simulink model "digiex3"  (R2017b)
settings: Solver=ode23tb  StartTime=0.0  StopTime=15  RelTol=1e-3
values from neighbouring files (symbols this model uses):
  AT_gain = ones(1,N)    [parameter_project.m]
  ctrl_mtrx2 = combvec(ctrl_mtrx',ctrl_mtrx')'    [parameter_project.m]
  DFCU_AT_REAL = DFCU.AT_Kv.*(1+0.2*(rand(1,N)-0.5))    [parameter_project.m]
  DFCU_PA_REAL = DFCU.PA_Kv.*(1+0.2*(rand(1,N)-0.5))    [parameter_project.m]
  Kff = 1    [User_interface.m]
  Kp = 10    [User_interface.m]
  Kv = 2.5e-7    (= 2.5e-07)    [parameter_project.m]
  PA_gain = ones(1,N)    [parameter_project.m]
  ptr = 1e5    (= 100000)    [parameter_project.m]
  switch_gain = 5e-2    (= 0.05)    [User_interface.m]
  ts = 0.01    [parameter_project.m]
undefined symbols (not defined in the file or in its folder): Controller, Cyl, DFCU, Fric, Load, Supply, Tank, Valve
libraries: dspmtrx3 x2, dspstat3 x1
settings Model: Creator=ganguly  LastModifiedBy=pallab
settings CodeAppCC: StateflowObjectComments=on
settings SimscapeCC: SimscapeNormalizeSystem=off

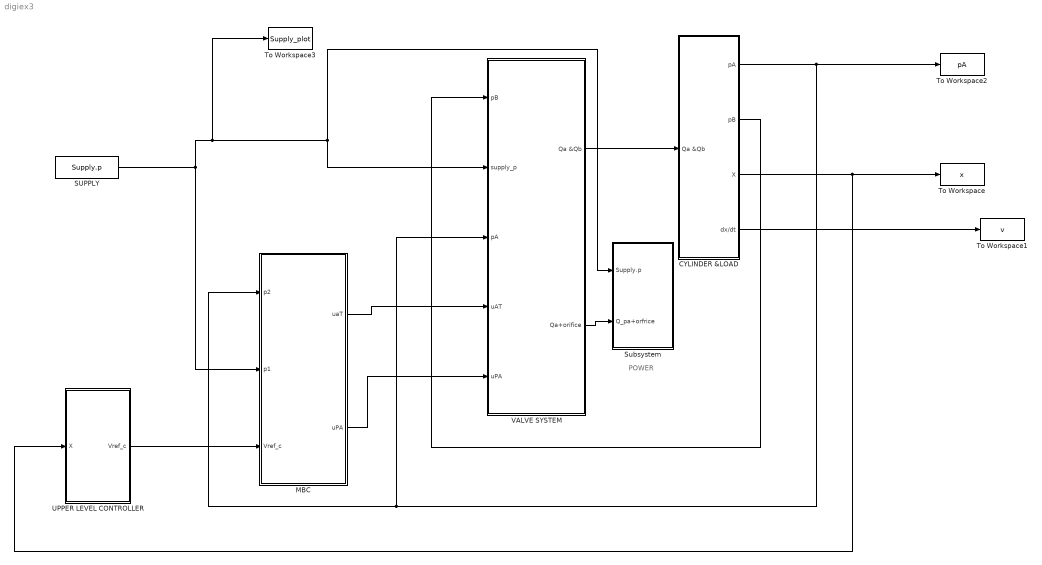
== system digiex3 ==
  note: POWER
  CYLINDER &LOAD : Subsystem
  MBC : Subsystem
  SUPPLY : Constant  Value=Supply.p
  Subsystem : Subsystem
  To Workspace : ToWorkspace  VariableName=x  SampleTime=-1
  To Workspace1 : ToWorkspace  VariableName=v  SampleTime=-1
  To Workspace2 : ToWorkspace  VariableName=pA  SampleTime=-1
  To Workspace3 : ToWorkspace  VariableName=Supply_plot  SampleTime=-1
      settings: Save2DSignal=2-D array (concatenate along first dimension)
  UPPER LEVEL CONTROLLER : Subsystem
  VALVE SYSTEM : Subsystem
  wires:
  SUPPLY/1 -> MBC/2(p1), To Workspace3/1, VALVE SYSTEM/2(supply_p), Subsystem/1(Supply.p)
  UPPER LEVEL CONTROLLER/1(Vref_c) -> MBC/3(Vref_c)
  CYLINDER &LOAD/3(X) -> UPPER LEVEL CONTROLLER/1(X), To Workspace/1
  CYLINDER &LOAD/1(pA) -> MBC/1(p2), VALVE SYSTEM/3(pA), To Workspace2/1
  VALVE SYSTEM/1(Qa &Qb) -> CYLINDER &LOAD/1(Qa &Qb)
  CYLINDER &LOAD/2(pB) -> VALVE SYSTEM/1(pB)
  CYLINDER &LOAD/4(dx/dt) -> To Workspace1/1
  MBC/2(uPA) -> VALVE SYSTEM/5(uPA)
  MBC/1(uaT) -> VALVE SYSTEM/4(uAT)
  VALVE SYSTEM/2(Qa+orifice) -> Subsystem/2(Q_pa+orfrice)

== system digiex3/CYLINDER &LOAD ==
  Qa &Qb : Inport
  Cylinder : Subsystem  mask(Hydraulic){D=[Cyl.D Cyl.d], xmax=Cyl.x_max, Vdead=[1e-4  1e-4], Vhose=[0 0], B_o=Cyl.B, Bhose=[400e6 400e6], pini=[Cyl.pA_init   Cyl.pB_init]}
      mask prompts: D "Diameters of piston and piston rod [m  m] :"; xmax "Cylindes stroke [m] :"; Vdead "Dead volumes at cylinder ends [m^3  m^3] :"; Vhose "Volumes of hoses [m^3  m^3] :"; B_o "Bulk modulus of oil [Pa] :"; Bhose "Bulk moduli of hoses [Pa  Pa] :"; pini "Initial pressures [Pa Pa] :"
      mask init:
      | A_A = pi/4*D(1)^2; A_B = A_A-pi/4*D(2)^2; V_0A = Vdead(1); V_0B = Vdead(2); V_HA = Vhose(1); V_HB = Vhose(2); B_HA = Bhose(1); B_HB = Bhose(2); p_0A = pini(1); p_0B = pini(2);
  Demux : Demux  Outputs=2
  Single mass model with friction and ends : Subsystem  mask(Mechanism){m=Load.m, range=[0, Cyl.x_max], xini=Cyl.x_init, Fricparams=[Fric.Fs  Fric.Fc  Fric.b  Fric.vtol Fric.m_est], presl=Fric.preslide, Kj=Cyl.End_K, g=-9.8}
      mask prompts: m "Mass [kg] :"; range "Range of motion [m  m] :"; xini "Initial position [m] :"; Fricparams "Friction parameters [Fs, Fc, b, vtol, mest]:"; presl "Pre-sliding displacement [m] :"; Kj "Spring constant of end [N/m] :"; g "gravity [m/s^2]"
      mask help:
      | Mechanism for linear movenment.
      | Model includes:
      | Inertia: F = m*a
      | Friction: Dynamic friction model (cf.IHA-2600)
      | End Springs: Use high spring constant and stiff solver for realistic results
      | Gravity: 0 if horizontal path, g if vertical. Careful with sign! (Look under mask)
      mask init:
      | xmax=range(2);xmin=range(1);
  pA : Outport
  pB : Outport  Port=2
  X : Outport  Port=3
  dx/dt : Outport  Port=4
  wires:
  Single mass model with friction and ends/1(x) -> X/1, Cylinder/2(x)
  Qa &Qb/1 -> Cylinder/1(QA & QB)
  Demux/2 -> pB/1
  Single mass model with friction and ends/2(dx/dt) -> dx/dt/1, Cylinder/3(dx/dt)
  Cylinder/1(pA & pB) -> Demux/1
  Cylinder/2(F) -> Single mass model with friction and ends/1(F)
  Demux/1 -> pA/1

== system digiex3/MBC ==
  p2 : Inport
  p1 : Inport  Port=2
  Vref_c : Inport  Port=3
  Constant1 : Constant  Value=Tank.p
  Gain2 : Gain  Gain=Cyl.area
  Gain4 : Gain  Gain=1/Cyl.area
  To Workspace : ToWorkspace  VariableName=v_est  SampleTime=-1
      settings: Save2DSignal=2-D array (concatenate along first dimension)
  mbc_PA : Subsystem
  uaT : Outport
  uPA : Outport  Port=2
  wires:
  mbc_PA/1(Q_estimate) -> Gain4/1
  p2/1 -> mbc_PA/3(pA1)
  Gain2/1 -> mbc_PA/1(Q_ref)
  mbc_PA/3(uaT) -> uaT/1
  Gain4/1 -> To Workspace/1
  mbc_PA/2(uPA) -> uPA/1
  p1/1 -> mbc_PA/2(pP)
  Vref_c/1 -> mbc_PA/5(V_ref), Gain2/1
  Constant1/1 -> mbc_PA/4(pT)

== system digiex3/Subsystem ==
  Supply.p : Inport
  Q_pa+orfrice : Inport  Port=2
  Gain1 : Gain  Gain=-1
  Product : Product
  To Workspace : ToWorkspace  VariableName=power  SampleTime=-1
  wires:
  Q_pa+orfrice/1 -> Product/2
  Supply.p/1 -> Product/1
  Product/1 -> Gain1/1
  Gain1/1 -> To Workspace/1

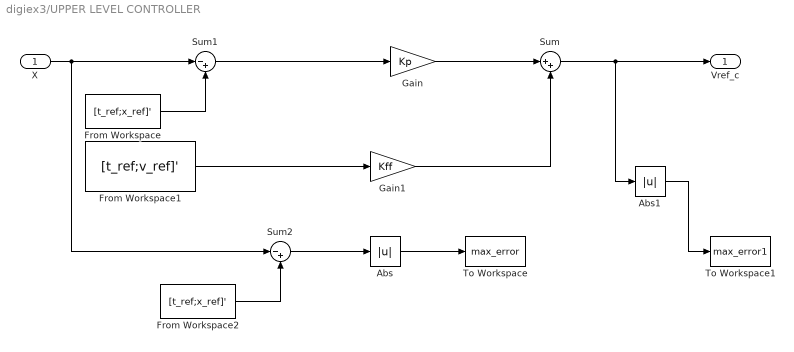
== system digiex3/UPPER LEVEL CONTROLLER ==
  X : Inport
  Abs : Abs
  Abs1 : Abs
  From Workspace : FromWorkspace  VariableName=[t_ref;x_ref]'  SampleTime=ts
  From Workspace1 : FromWorkspace  VariableName=[t_ref;v_ref]'  SampleTime=ts
  From Workspace2 : FromWorkspace  VariableName=[t_ref;x_ref]'  SampleTime=ts
  Gain : Gain  Gain=Kp
  Gain1 : Gain  Gain=Kff
  Sum : Sum  Inputs=|++
  Sum1 : Sum  Inputs=|-+
  Sum2 : Sum  Inputs=|-+
  To Workspace : ToWorkspace  VariableName=max_error  SampleTime=-1
  To Workspace1 : ToWorkspace  VariableName=max_error1  SampleTime=-1
  Vref_c : Outport
  wires:
  From Workspace/1 -> Sum1/2
  Sum1/1 -> Gain/1
  Gain1/1 -> Sum/2
  Gain/1 -> Sum/1
  From Workspace1/1 -> Gain1/1
  Sum2/1 -> Abs/1
  From Workspace2/1 -> Sum2/2
  X/1 -> Sum2/1, Sum1/1
  Abs/1 -> To Workspace/1
  Sum/1 -> Abs1/1, Vref_c/1
  Abs1/1 -> To Workspace1/1

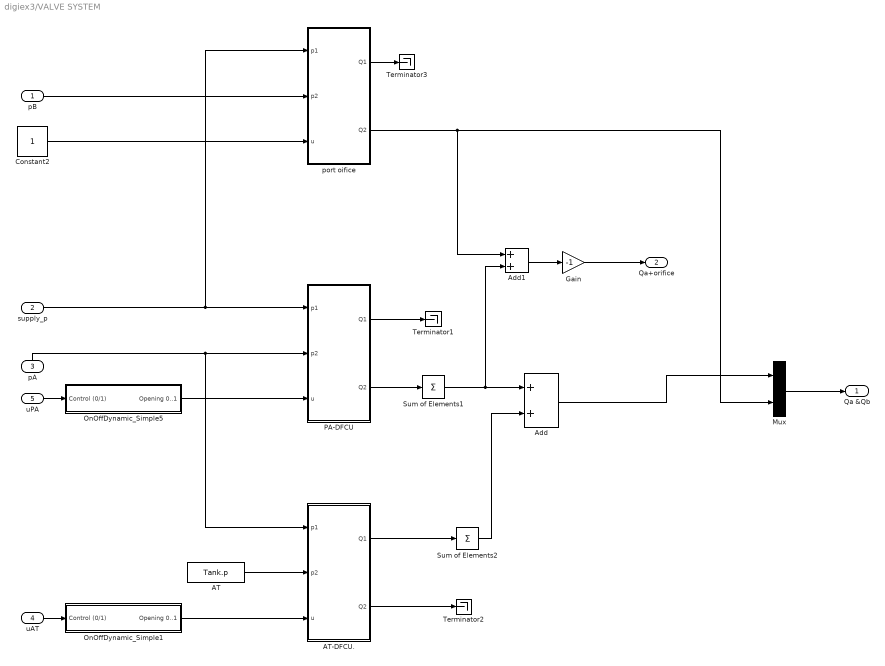
== system digiex3/VALVE SYSTEM ==
  pB : Inport
  supply_p : Inport  Port=2
  pA : Inport  Port=3
  uAT : Inport  Port=4
  uPA : Inport  Port=5
  AT : Constant  Value=Tank.p
  "AT-DFCU. " : Subsystem  TreatAsAtomicUnit=on  mask(Hydraulics){Kv=DFCU_AT_REAL, ptr=ptr}
      mask prompts: Kv "Orifice Flow Coefficient [SI-units]:"; ptr "Transition pressure [Pa] :"
      mask help:
      | Implements numerically robust turbulent flow equation. Square root model during turbulent flow.
      | Polynomial flow equation is used when abs(dp) is smaller than transition pressure.
      | [Source: Ellman, A. & Piche, R. 1996.
      | A Modified Orifice Flow Formula for Numerical Simulation of Fluid Power Systems.
      | Fluid Power Systems and Technology, ASME]
      |
      | Modified for Digital Hydraulics:
      | Use scalar parameters model on/off-valve.
      | Use vector parameters model array of on/off-valves a.k.a DFCU
  Add : Sum
  Add1 : Sum
  Constant2 : Constant
  Gain : Gain  Gain=-1
  Mux : Mux  Inputs=2
  OnOffDynamic_Simple1 : Subsystem  TreatAsAtomicUnit=on  mask(Digital Hydraulics){delay_open=Valve.switch_o_delay, delay_close=Valve.switch_c_delay, time_open=Valve.switch_o_time, time_close=Valve.switch_c_time}
      mask prompts: delay_open "Opening delay"; delay_close "Closing delay"; time_open "Opening switch time"; time_close "Closing switch time"
      mask help:
      | Simple dynamics. For on/off-valves only.
      |
      | Models valve switching dynamics with delay and limited armature
      | movenment speed. Modelled to have low computational cost but good enoug
      | accuracy.
      |
      | Model is valid for:
      | -Controller testing, PCM, PNM, etc.
      | -State transition inspection*
      | -Fault tolerance testing
      | -Low frequency PWM
      |
      | Model is NOT valid for:
      | -Control styles utilizing frequencies higher than on/off-valve operational
      | frequency.
      | -Ballistic mode
      | -Proportional valves
      |
      | *NOTE!
      | Delay can be eihter scalar or vector, but movenment time must be scalar or
      | something does not work properly. If delay is scalar, same delay is used for
      | all signals.
      mask init:
      | Opening_delay = delay_open;
      | Closing_delay = delay_close;
      | Opening_slew = 1/time_open;
      | Closing_slew = -1/time_close;
  OnOffDynamic_Simple5 : Subsystem  TreatAsAtomicUnit=on  mask(Digital Hydraulics){delay_open=Valve.switch_o_delay, delay_close=Valve.switch_c_delay, time_open=Valve.switch_o_time, time_close=Valve.switch_c_time}
      mask prompts: delay_open "Opening delay"; delay_close "Closing delay"; time_open "Opening switch time"; time_close "Closing switch time"
      mask help:
      | Simple dynamics. For on/off-valves only.
      |
      | Models valve switching dynamics with delay and limited armature
      | movenment speed. Modelled to have low computational cost but good enoug
      | accuracy.
      |
      | Model is valid for:
      | -Controller testing, PCM, PNM, etc.
      | -State transition inspection*
      | -Fault tolerance testing
      | -Low frequency PWM
      |
      | Model is NOT valid for:
      | -Control styles utilizing frequencies higher than on/off-valve operational
      | frequency.
      | -Ballistic mode
      | -Proportional valves
      |
      | *NOTE!
      | Delay can be eihter scalar or vector, but movenment time must be scalar or
      | something does not work properly. If delay is scalar, same delay is used for
      | all signals.
      mask init:
      | Opening_delay = delay_open;
      | Closing_delay = delay_close;
      | Opening_slew = 1/time_open;
      | Closing_slew = -1/time_close;
  PA-DFCU : Subsystem  TreatAsAtomicUnit=on  mask(Hydraulics){Kv=DFCU_PA_REAL, ptr=ptr}
      mask prompts: Kv "Orifice Flow Coefficient [SI-units]:"; ptr "Transition pressure [Pa] :"
      mask help:
      | Implements numerically robust turbulent flow equation. Square root model during turbulent flow.
      | Polynomial flow equation is used when abs(dp) is smaller than transition pressure.
      | [Source: Ellman, A. & Piche, R. 1996.
      | A Modified Orifice Flow Formula for Numerical Simulation of Fluid Power Systems.
      | Fluid Power Systems and Technology, ASME]
      |
      | Modified for Digital Hydraulics:
      | Use scalar parameters model on/off-valve.
      | Use vector parameters model array of on/off-valves a.k.a DFCU
  Sum of Elements1 : Sum  Inputs=+
  Sum of Elements2 : Sum  Inputs=+
  Terminator1 : Terminator
  Terminator2 : Terminator
  Terminator3 : Terminator
  port oifice : Subsystem  TreatAsAtomicUnit=on  mask(Hydraulics){Kv=Kv, ptr=ptr}
      mask prompts: Kv "Orifice Flow Coefficient [SI-units]:"; ptr "Transition pressure [Pa] :"
      mask help:
      | Implements numerically robust turbulent flow equation. Square root model during turbulent flow.
      | Polynomial flow equation is used when abs(dp) is smaller than transition pressure.
      | [Source: Ellman, A. & Piche, R. 1996.
      | A Modified Orifice Flow Formula for Numerical Simulation of Fluid Power Systems.
      | Fluid Power Systems and Technology, ASME]
      |
      | Modified for Digital Hydraulics:
      | Use scalar parameters model on/off-valve.
      | Use vector parameters model array of on/off-valves a.k.a DFCU
  Qa &Qb : Outport
  Qa+orifice : Outport  Port=2
  wires:
  pA/1 -> "AT-DFCU. "/1(p1), PA-DFCU/2(p2)
  supply_p/1 -> port oifice/1(p1), PA-DFCU/1(p1)
  PA-DFCU/2(Q2) -> Sum of Elements1/1
  PA-DFCU/1(Q1) -> Terminator1/1
  "AT-DFCU. "/1(Q1) -> Sum of Elements2/1
  "AT-DFCU. "/2(Q2) -> Terminator2/1
  AT/1 -> "AT-DFCU. "/2(p2)
  Constant2/1 -> port oifice/3(u)
  Mux/1 -> Qa &Qb/1
  pB/1 -> port oifice/2(p2)
  port oifice/1(Q1) -> Terminator3/1
  uAT/1 -> OnOffDynamic_Simple1/1(Control (0/1))
  Sum of Elements2/1 -> Add/2
  Sum of Elements1/1 -> Add1/2, Add/1
  uPA/1 -> OnOffDynamic_Simple5/1(Control (0/1))
  Add/1 -> Mux/1
  port oifice/2(Q2) -> Add1/1, Mux/2
  OnOffDynamic_Simple1/1(Opening 0..1) -> "AT-DFCU. "/3(u)
  OnOffDynamic_Simple5/1(Opening 0..1) -> PA-DFCU/3(u)
  Add1/1 -> Gain/1
  Gain/1 -> Qa+orifice/1

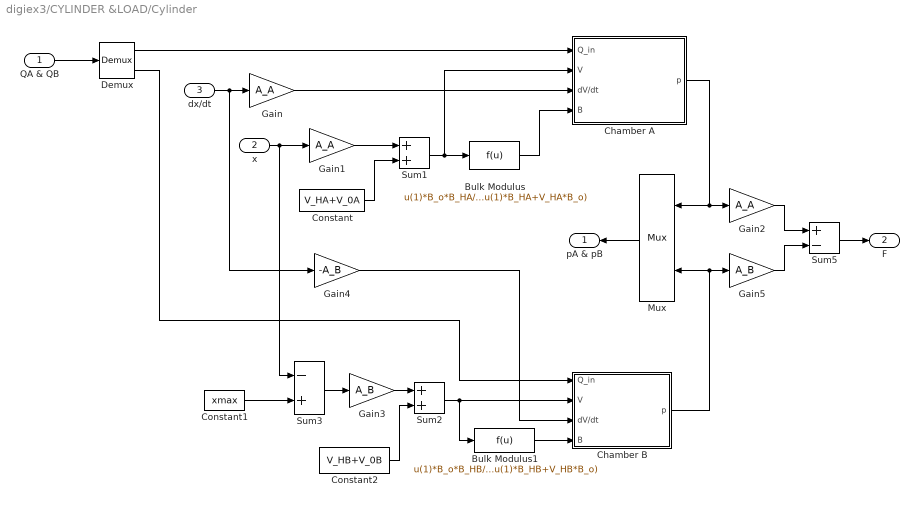
== system digiex3/CYLINDER &LOAD/Cylinder ==
  QA & QB : Inport
  x : Inport  Port=2
  dx/dt : Inport  Port=3
  Bulk Modulus : Fcn  Expr=u(1)*B_o*B_HA/(u(1)*B_HA+V_HA*B_o)
  Bulk Modulus1 : Fcn  Expr=u(1)*B_o*B_HB/(u(1)*B_HB+V_HB*B_o)
  Chamber A : Subsystem  mask(Hydraulic){pinitial=p_0A}
      mask prompts: pinitial "Initial pressure [Pa] :"
      mask help: Lumped fluid volume. Pressure is limited greater or equal to zero by saturation block corresponding to a rough model of cavitation.
      mask Help: eval('hydlibdoc(''vol_cav_doc'')')
  Chamber B : Subsystem  mask(Hydraulic){pinitial=p_0B}
      mask prompts: pinitial "Initial pressure [Pa] :"
      mask help: Lumped fluid volume. Pressure is limited greater or equal to zero by saturation block corresponding to a rough model of cavitation.
      mask Help: eval('hydlibdoc(''vol_cav_doc'')')
  Constant : Constant  Value=V_HA+V_0A
  Constant1 : Constant  Value=xmax
  Constant2 : Constant  Value=V_HB+V_0B
  Demux : Demux  Outputs=2
  Gain : Gain  Gain=A_A  SaturateOnIntegerOverflow=on  OutDataTypeStr=Inherit: Same as input  ParamDataTypeStr=Inherit: Same as input
  Gain1 : Gain  Gain=A_A  SaturateOnIntegerOverflow=on  OutDataTypeStr=Inherit: Same as input  ParamDataTypeStr=Inherit: Same as input
  Gain2 : Gain  Gain=A_A  SaturateOnIntegerOverflow=on  OutDataTypeStr=Inherit: Same as input  ParamDataTypeStr=Inherit: Same as input
  Gain3 : Gain  Gain=A_B  SaturateOnIntegerOverflow=on  OutDataTypeStr=Inherit: Same as input  ParamDataTypeStr=Inherit: Same as input
  Gain4 : Gain  Gain=-A_B  SaturateOnIntegerOverflow=on  OutDataTypeStr=Inherit: Same as input  ParamDataTypeStr=Inherit: Same as input
  Gain5 : Gain  Gain=A_B  SaturateOnIntegerOverflow=on  OutDataTypeStr=Inherit: Same as input  ParamDataTypeStr=Inherit: Same as input
  Mux : Mux  Inputs=2
  Sum1 : Sum  SaturateOnIntegerOverflow=on  InputSameDT=on  OutDataTypeStr=Inherit: Same as first input
  Sum2 : Sum  SaturateOnIntegerOverflow=on  InputSameDT=on  OutDataTypeStr=Inherit: Same as first input
  Sum3 : Sum  Inputs=-+  SaturateOnIntegerOverflow=on  InputSameDT=on  OutDataTypeStr=Inherit: Same as first input
  Sum5 : Sum  Inputs=+-  SaturateOnIntegerOverflow=on  InputSameDT=on  OutDataTypeStr=Inherit: Same as first input
  pA & pB : Outport  InitialOutput=0
  F : Outport  Port=2  InitialOutput=0
  wires:
  Constant/1 -> Sum1/2
  Sum1/1 -> Chamber A/2(" V"), Bulk Modulus/1
  Gain1/1 -> Sum1/1
  x/1 -> Gain1/1, Sum3/1
  QA & QB/1 -> Demux/1
  Chamber B/1(p) -> Gain5/1, Mux/2
  Sum5/1 -> F/1
  Gain5/1 -> Sum5/2
  Gain2/1 -> Sum5/1
  Chamber A/1(p) -> Gain2/1, Mux/1
  Mux/1 -> pA & pB/1
  Bulk Modulus/1 -> Chamber A/4(" B")
  Demux/1 -> Chamber A/1(Q_in)
  Bulk Modulus1/1 -> Chamber B/4(" B")
  Gain4/1 -> Chamber B/3(" dV/dt")
  Sum2/1 -> Chamber B/2(" V"), Bulk Modulus1/1
  Demux/2 -> Chamber B/1(Q_in)
  Constant1/1 -> Sum3/2
  Sum3/1 -> Gain3/1
  Gain3/1 -> Sum2/1
  Constant2/1 -> Sum2/2
  Gain/1 -> Chamber A/3(" dV/dt")
  dx/dt/1 -> Gain/1, Gain4/1

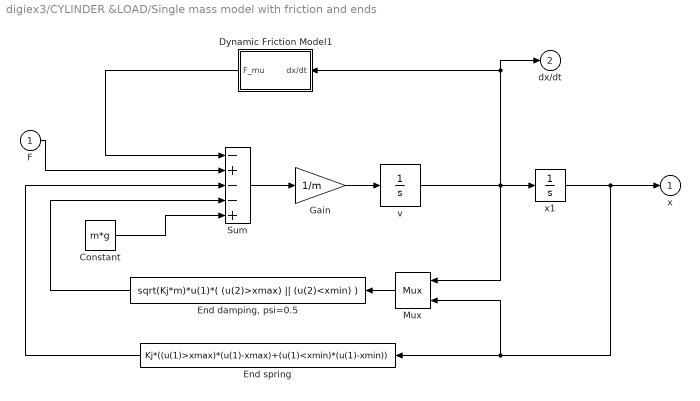
== system digiex3/CYLINDER &LOAD/Single mass model with friction and ends ==
  F : Inport
  Constant : Constant  Value=m*g
  Dynamic Friction Model1 : Subsystem  mask(Mechanic){Fs=Fricparams(1), Fc=Fricparams(2), b=Fricparams(3), vtol=Fricparams(4), presl=presl, mest=Fricparams(5)}
      mask prompts: Fs "Static friction force [N] :"; Fc "Coulombic friction force [N] :"; b "Coefficient of viscous friction [Ns/m]:"; vtol "Velocity of minimum friction force [m/s] :"; presl "Pre-sliding displacement [m] :"; mest "Estimate of load mass [kg] :"
      mask init:
      | sigma0 = Fs/presl; sigma1 = 2*sqrt(sigma0*mest);
  "End damping, psi=0.5" : Fcn  Expr=sqrt(Kj*m)*u(1)*( (u(2)>xmax) || (u(2)<xmin) )
  End spring : Fcn  Expr=Kj*((u(1)>xmax)*(u(1)-xmax)+(u(1)<xmin)*(u(1)-xmin))
  Gain : Gain  Gain=1/m  SaturateOnIntegerOverflow=on  OutDataTypeStr=Inherit: Same as input  ParamDataTypeStr=Inherit: Same as input
  Mux : Mux  Inputs=2
  Sum : Sum  Inputs=-+--+  SaturateOnIntegerOverflow=on  InputSameDT=on  OutDataTypeStr=Inherit: Same as first input
  v : Integrator
  x1 : Integrator  InitialCondition=xini
  x : Outport  InitialOutput=0
  dx/dt : Outport  Port=2  InitialOutput=0
  wires:
  v/1 -> Mux/1, x1/1, Dynamic Friction Model1/1(dx/dt), dx/dt/1
  Mux/1 -> "End damping, psi=0.5"/1
  "End damping, psi=0.5"/1 -> Sum/4
  End spring/1 -> Sum/3
  Sum/1 -> Gain/1
  Gain/1 -> v/1
  x1/1 -> Mux/2, End spring/1, x/1
  Dynamic Friction Model1/1(F_mu) -> Sum/1
  F/1 -> Sum/2
  Constant/1 -> Sum/5

== system digiex3/MBC/mbc_PA ==
  note: STATE
  note: CONTROL MATRIX
  note: SWITCH_COST
  note: MINIMUM
  Q_ref : Inport
  pP : Inport  Port=2
  pA1 : Inport  Port=3
  pT : Inport  Port=4
  V_ref : Inport  Port=5
  "CROSS FLOW " : Subsystem
  SUM FLOW CONTROLLER : Subsystem
  SWITCHING COST : Subsystem
  Q_estimate : Outport
  uPA : Outport  Port=2
  uaT : Outport  Port=3
  wires:
  SUM FLOW CONTROLLER/5(Control_matrix) -> SWITCHING COST/2(CONTROL_MATRIX)
  SWITCHING COST/1(MINIMUM) -> SUM FLOW CONTROLLER/5(Min)
  SUM FLOW CONTROLLER/6(Con_PA) -> "CROSS FLOW "/1(CONTROL_PA)
  pT/1 -> SUM FLOW CONTROLLER/4(pT)
  SUM FLOW CONTROLLER/2(uPA) -> uPA/1
  "CROSS FLOW "/1(SECONDARY COST) -> SUM FLOW CONTROLLER/6(Switch_cost)
  SUM FLOW CONTROLLER/8(Q_PA) -> "CROSS FLOW "/4(Q_PA-)
  V_ref/1 -> "CROSS FLOW "/3(v)
  SUM FLOW CONTROLLER/3(uaT) -> uaT/1
  SUM FLOW CONTROLLER/1(Q_estimate) -> Q_estimate/1
  SUM FLOW CONTROLLER/9(Q_AT) -> "CROSS FLOW "/5(Q_AT)
  SUM FLOW CONTROLLER/4(State) -> SWITCHING COST/1(STATE)
  SUM FLOW CONTROLLER/7(Con_AT) -> "CROSS FLOW "/2(CONTROL_AT)
  pA1/1 -> SUM FLOW CONTROLLER/3(pA1)
  Q_ref/1 -> SUM FLOW CONTROLLER/2(Q_ref)
  pP/1 -> SUM FLOW CONTROLLER/1(pP)

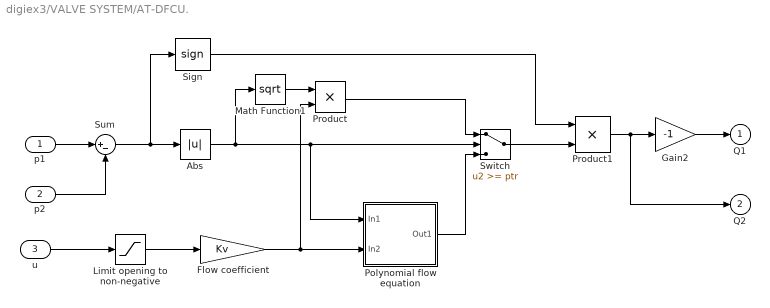
== system digiex3/VALVE SYSTEM/AT-DFCU.  ==
  p1 : Inport
  p2 : Inport  Port=2
  u : Inport  Port=3
  Abs : Abs  ZeroCross=off  SaturateOnIntegerOverflow=on
  Flow coefficient : Gain  Gain=Kv  SaturateOnIntegerOverflow=on  OutDataTypeStr=Inherit: Same as input  ParamDataTypeStr=Inherit: Same as input
  Gain2 : Gain  Gain=-1  SaturateOnIntegerOverflow=on  OutDataTypeStr=Inherit: Same as input  ParamDataTypeStr=Inherit: Same as input
  Limit opening to non-negative : Saturate  UpperLimit=inf  LowerLimit=0
  Math Function1 : Math  Operator=sqrt  SaturateOnIntegerOverflow=on
  Polynomial flow equation : Subsystem
  Product : Product  SaturateOnIntegerOverflow=on  InputSameDT=on  OutDataTypeStr=Inherit: Same as first input
  Product1 : Product  SaturateOnIntegerOverflow=on  InputSameDT=on  OutDataTypeStr=Inherit: Same as first input
  Sign : Signum  ZeroCross=off
  Sum : Sum  Inputs=|+-
  Switch : Switch  Threshold=ptr  ZeroCross=off  SaturateOnIntegerOverflow=on  InputSameDT=on
  Q1 : Outport  InitialOutput=0
  Q2 : Outport  Port=2  InitialOutput=0
  wires:
  Gain2/1 -> Q1/1
  u/1 -> Limit opening to non-negative/1
  Sum/1 -> Abs/1, Sign/1
  Polynomial flow equation/1(Out1) -> Switch/3
  Product/1 -> Switch/1
  Math Function1/1 -> Product/1
  Abs/1 -> Switch/2, Polynomial flow equation/1(In1), Math Function1/1
  Limit opening to non-negative/1 -> Flow coefficient/1
  Flow coefficient/1 -> Product/2, Polynomial flow equation/2(In2)
  Sign/1 -> Product1/1
  Product1/1 -> Q2/1, Gain2/1
  Switch/1 -> Product1/2
  p1/1 -> Sum/1
  p2/1 -> Sum/2

== system digiex3/VALVE SYSTEM/OnOffDynamic_Simple1 ==
  Control (0/1) : Inport
  Closing delay : TransportDelay  DelayTime=Closing_delay
  Opening delay : TransportDelay  DelayTime=Opening_delay
  Rate Limiter : RateLimiter  RisingSlewLimit=Opening_slew  FallingSlewLimit=Closing_slew  SampleTimeMode=inherited
  Switch : Switch  Threshold=0.5
  Opening 0..1 : Outport
  wires:
  Switch/1 -> Rate Limiter/1
  Closing delay/1 -> Switch/3
  Control (0/1)/1 -> Closing delay/1, Switch/2, Opening delay/1
  Opening delay/1 -> Switch/1
  Rate Limiter/1 -> Opening 0..1/1

== system digiex3/VALVE SYSTEM/OnOffDynamic_Simple5 ==
  Control (0/1) : Inport
  Closing delay : TransportDelay  DelayTime=Closing_delay
  Opening delay : TransportDelay  DelayTime=Opening_delay
  Rate Limiter : RateLimiter  RisingSlewLimit=Opening_slew  FallingSlewLimit=Closing_slew  SampleTimeMode=inherited
  Switch : Switch  Threshold=0.5
  Opening 0..1 : Outport
  wires:
  Rate Limiter/1 -> Opening 0..1/1
  Opening delay/1 -> Switch/1
  Control (0/1)/1 -> Opening delay/1, Switch/2, Closing delay/1
  Closing delay/1 -> Switch/3
  Switch/1 -> Rate Limiter/1

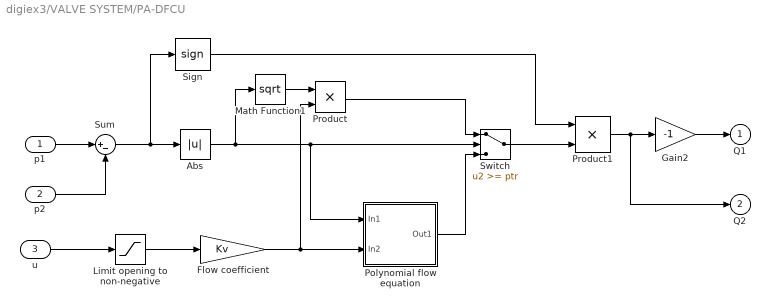
== system digiex3/VALVE SYSTEM/PA-DFCU ==
  p1 : Inport
  p2 : Inport  Port=2
  u : Inport  Port=3
  Abs : Abs  ZeroCross=off  SaturateOnIntegerOverflow=on
  Flow coefficient : Gain  Gain=Kv  SaturateOnIntegerOverflow=on  OutDataTypeStr=Inherit: Same as input  ParamDataTypeStr=Inherit: Same as input
  Gain2 : Gain  Gain=-1  SaturateOnIntegerOverflow=on  OutDataTypeStr=Inherit: Same as input  ParamDataTypeStr=Inherit: Same as input
  Limit opening to non-negative : Saturate  UpperLimit=inf  LowerLimit=0
  Math Function1 : Math  Operator=sqrt  SaturateOnIntegerOverflow=on
  Polynomial flow equation : Subsystem
  Product : Product  SaturateOnIntegerOverflow=on  InputSameDT=on  OutDataTypeStr=Inherit: Same as first input
  Product1 : Product  SaturateOnIntegerOverflow=on  InputSameDT=on  OutDataTypeStr=Inherit: Same as first input
  Sign : Signum  ZeroCross=off
  Sum : Sum  Inputs=|+-
  Switch : Switch  Threshold=ptr  ZeroCross=off  SaturateOnIntegerOverflow=on  InputSameDT=on
  Q1 : Outport  InitialOutput=0
  Q2 : Outport  Port=2  InitialOutput=0
  wires:
  p2/1 -> Sum/2
  p1/1 -> Sum/1
  Switch/1 -> Product1/2
  Product1/1 -> Gain2/1, Q2/1
  Sign/1 -> Product1/1
  Flow coefficient/1 -> Polynomial flow equation/2(In2), Product/2
  Limit opening to non-negative/1 -> Flow coefficient/1
  Abs/1 -> Math Function1/1, Polynomial flow equation/1(In1), Switch/2
  Math Function1/1 -> Product/1
  Product/1 -> Switch/1
  Polynomial flow equation/1(Out1) -> Switch/3
  Sum/1 -> Sign/1, Abs/1
  u/1 -> Limit opening to non-negative/1
  Gain2/1 -> Q1/1

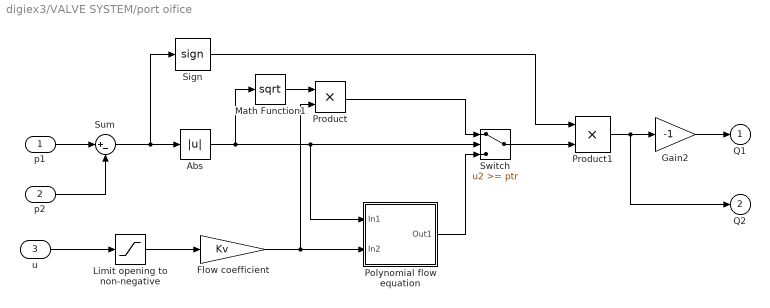
== system digiex3/VALVE SYSTEM/port oifice ==
  p1 : Inport
  p2 : Inport  Port=2
  u : Inport  Port=3
  Abs : Abs  ZeroCross=off  SaturateOnIntegerOverflow=on
  Flow coefficient : Gain  Gain=Kv  SaturateOnIntegerOverflow=on  OutDataTypeStr=Inherit: Same as input  ParamDataTypeStr=Inherit: Same as input
  Gain2 : Gain  Gain=-1  SaturateOnIntegerOverflow=on  OutDataTypeStr=Inherit: Same as input  ParamDataTypeStr=Inherit: Same as input
  Limit opening to non-negative : Saturate  UpperLimit=inf  LowerLimit=0
  Math Function1 : Math  Operator=sqrt  SaturateOnIntegerOverflow=on
  Polynomial flow equation : Subsystem
  Product : Product  SaturateOnIntegerOverflow=on  InputSameDT=on  OutDataTypeStr=Inherit: Same as first input
  Product1 : Product  SaturateOnIntegerOverflow=on  InputSameDT=on  OutDataTypeStr=Inherit: Same as first input
  Sign : Signum  ZeroCross=off
  Sum : Sum  Inputs=|+-
  Switch : Switch  Threshold=ptr  ZeroCross=off  SaturateOnIntegerOverflow=on  InputSameDT=on
  Q1 : Outport  InitialOutput=0
  Q2 : Outport  Port=2  InitialOutput=0
  wires:
  p2/1 -> Sum/2
  p1/1 -> Sum/1
  Switch/1 -> Product1/2
  Product1/1 -> Gain2/1, Q2/1
  Sign/1 -> Product1/1
  Flow coefficient/1 -> Polynomial flow equation/2(In2), Product/2
  Limit opening to non-negative/1 -> Flow coefficient/1
  Abs/1 -> Math Function1/1, Polynomial flow equation/1(In1), Switch/2
  Math Function1/1 -> Product/1
  Product/1 -> Switch/1
  Polynomial flow equation/1(Out1) -> Switch/3
  Sum/1 -> Sign/1, Abs/1
  u/1 -> Limit opening to non-negative/1
  Gain2/1 -> Q1/1

== system digiex3/CYLINDER &LOAD/Cylinder/Chamber A ==
  Q_in : Inport
  " V" : Inport  Port=2
  " dV/dt" : Inport  Port=3
  " B" : Inport  Port=4
  Integrator : Integrator  InitialCondition=pinitial  AbsoluteTolerance=10
  Product : Product  Inputs=*/*  SaturateOnIntegerOverflow=on  InputSameDT=on  OutDataTypeStr=Inherit: Same as first input
  Saturation : Saturate  UpperLimit=inf  LowerLimit=0
  Sum : Sum  Inputs=+-  SaturateOnIntegerOverflow=on  InputSameDT=on  OutDataTypeStr=Inherit: Same as first input
  p : Outport
  wires:
  Product/1 -> Integrator/1
  Integrator/1 -> Saturation/1
  Saturation/1 -> p/1
  " V"/1 -> Product/2
  " B"/1 -> Product/3
  Q_in/1 -> Sum/1
  " dV/dt"/1 -> Sum/2
  Sum/1 -> Product/1

== system digiex3/CYLINDER &LOAD/Cylinder/Chamber B ==
  Q_in : Inport
  " V" : Inport  Port=2
  " dV/dt" : Inport  Port=3
  " B" : Inport  Port=4
  Integrator : Integrator  InitialCondition=pinitial  AbsoluteTolerance=10
  Product : Product  Inputs=*/*  SaturateOnIntegerOverflow=on  InputSameDT=on  OutDataTypeStr=Inherit: Same as first input
  Saturation : Saturate  UpperLimit=inf  LowerLimit=0
  Sum : Sum  Inputs=+-  SaturateOnIntegerOverflow=on  InputSameDT=on  OutDataTypeStr=Inherit: Same as first input
  p : Outport
  wires:
  Product/1 -> Integrator/1
  Integrator/1 -> Saturation/1
  Saturation/1 -> p/1
  " V"/1 -> Product/2
  " B"/1 -> Product/3
  Q_in/1 -> Sum/1
  " dV/dt"/1 -> Sum/2
  Sum/1 -> Product/1

== system digiex3/CYLINDER &LOAD/Single mass model with friction and ends/Dynamic Friction Model1 ==
  dx/dt : Inport
  Abs : Abs  SaturateOnIntegerOverflow=on
  Fcn1 : Fcn  Expr=(Fc+(Fs-Fc)*exp(-u(1)*u(1)/vtol/vtol))/sigma0
  Gain3 : Gain  Gain=sigma0  SaturateOnIntegerOverflow=on  OutDataTypeStr=Inherit: Same as input  ParamDataTypeStr=Inherit: Same as input
  Gain4 : Gain  Gain=sigma1  SaturateOnIntegerOverflow=on  OutDataTypeStr=Inherit: Same as input  ParamDataTypeStr=Inherit: Same as input
  Integrator : Integrator
  Product : Product  Inputs=**/  SaturateOnIntegerOverflow=on  InputSameDT=on  OutDataTypeStr=Inherit: Same as first input
  Sum : Sum  Inputs=+-  SaturateOnIntegerOverflow=on  InputSameDT=on  OutDataTypeStr=Inherit: Same as first input
  Sum1 : Sum  Inputs=+++  SaturateOnIntegerOverflow=on  InputSameDT=on  OutDataTypeStr=Inherit: Same as first input
  Viskoosikitkakerroin : Gain  Gain=b  SaturateOnIntegerOverflow=on  OutDataTypeStr=Inherit: Same as input  ParamDataTypeStr=Inherit: Same as input
  F_mu : Outport
  wires:
  Integrator/1 -> Gain3/1, Product/1
  Sum1/1 -> F_mu/1
  Viskoosikitkakerroin/1 -> Sum1/3
  Sum/1 -> Gain4/1, Integrator/1
  dx/dt/1 -> Viskoosikitkakerroin/1, Abs/1, Fcn1/1, Sum/1
  Product/1 -> Sum/2
  Fcn1/1 -> Product/3
  Abs/1 -> Product/2
  Gain3/1 -> Sum1/2
  Gain4/1 -> Sum1/1

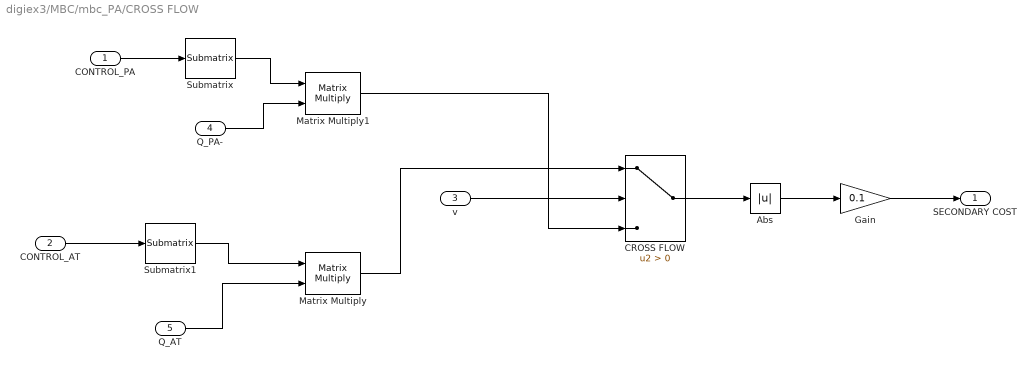
== system digiex3/MBC/mbc_PA/CROSS FLOW  ==
  CONTROL_PA : Inport
  CONTROL_AT : Inport  Port=2
  v : Inport  Port=3
  Q_PA- : Inport  Port=4
  Q_AT : Inport  Port=5
  Abs : Abs
  CROSS FLOW : Switch  Criteria=u2 > Threshold
  Gain : Gain  Gain=0.1
  Matrix Multiply : Product  Multiplication=Matrix(*)
  Matrix Multiply1 : Product  Multiplication=Matrix(*)
  Submatrix : dspmtrx3/Submatrix  RowSpan=Range of rows  RowStartMode=First  RowStartIndex=1  RowEndMode=Last  RowEndIndex=1  ColSpan=Range of columns  ColStartMode=First  ColStartIndex=1  ColEndMode=Offset from middle  ColEndIndex=-1
  Submatrix1 : dspmtrx3/Submatrix  RowSpan=Range of rows  RowStartMode=First  RowStartIndex=1  RowEndMode=Last  RowEndIndex=1  ColSpan=Range of columns  ColStartMode=Offset from middle  ColStartIndex=0  ColEndMode=Last  ColEndIndex=-1
  SECONDARY COST : Outport
  wires:
  CONTROL_AT/1 -> Submatrix1/1
  CONTROL_PA/1 -> Submatrix/1
  v/1 -> CROSS FLOW/2
  Submatrix1/1 -> Matrix Multiply/1
  Q_AT/1 -> Matrix Multiply/2
  Submatrix/1 -> Matrix Multiply1/1
  Q_PA-/1 -> Matrix Multiply1/2
  CROSS FLOW/1 -> Abs/1
  Gain/1 -> SECONDARY COST/1
  Abs/1 -> Gain/1
  Matrix Multiply/1 -> CROSS FLOW/1
  Matrix Multiply1/1 -> CROSS FLOW/3

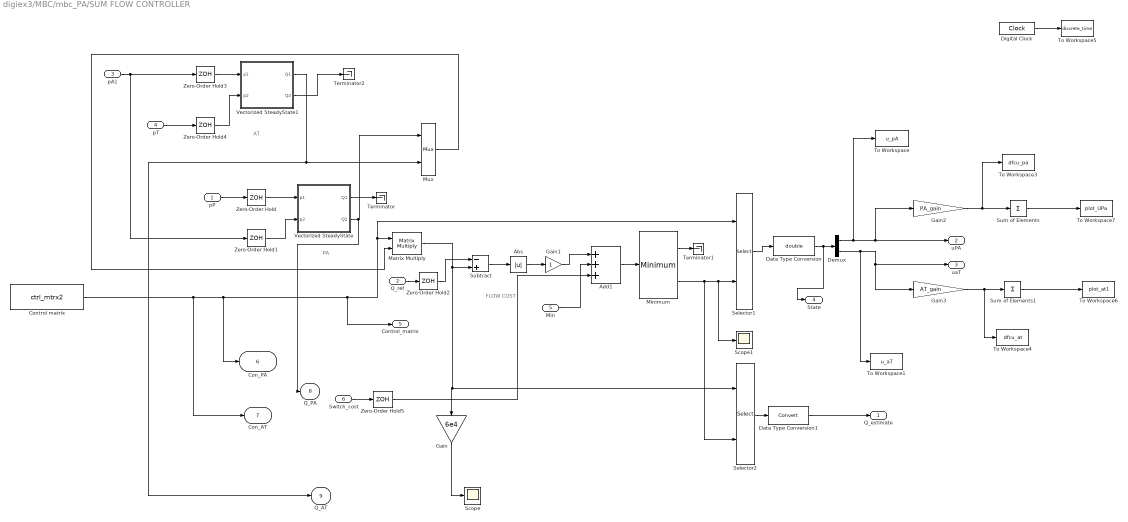
== system digiex3/MBC/mbc_PA/SUM FLOW CONTROLLER ==
  note: PA
  note: AT
  note: FLOW COST
  pP : Inport
  Q_ref : Inport  Port=2
  pA1 : Inport  Port=3
  pT : Inport  Port=4
  Min : Inport  Port=5
  Switch_cost : Inport  Port=6
  Abs : Abs
  Add1 : Sum  Inputs=+++
  Control matrix : Constant  Value=ctrl_mtrx2  SampleTime=Controller.ts
  Data Type Conversion : DataTypeConversion  OutDataTypeStr=double
  Data Type Conversion1 : DataTypeConversion
  Demux : Demux  Outputs=2
  Digital Clock : DigitalClock  SampleTime=Controller.ts
  Gain : Gain  Gain=6e4
  Gain1 : Gain
  Gain2 : Gain  Gain=PA_gain
  Gain3 : Gain  Gain=AT_gain
  Matrix Multiply : Product  Multiplication=Matrix(*)
  Minimum : dspstat3/Minimum  operation=minimum  fcn=Value and Index  indexBase=Zero  operateOver=Each column  Dimension=1  InputProcessing=Columns as channels (frame based)  reset=None  roiEnable=off  roiType=Rectangles  roiPortion=Entire ROI  roiOutput=Individual statistics for each ROI  roiFlag=off  roundingMode=Floor  overflowMode=off
      settings: SourceProductName=DSP System Toolbox  SourceProductBaseCode=DS
  Mux : Mux  Inputs=2
  Scope : Scope
  Scope1 : Scope
  Selector1 : Selector  NumberOfDimensions=2  IndexMode=Zero-based  InputPortWidth=3  IndexOptions=Index vector (port),Select all  Indices=[1 3],[1:2]  OutputSizes=1,1
  Selector2 : Selector  NumberOfDimensions=2  IndexMode=Zero-based  InputPortWidth=3  IndexOptions=Index vector (port),Select all  Indices=[1 3],[1:2]  OutputSizes=1,1
  Subtract : Sum  Inputs=-+
  Sum of Elements : Sum  Inputs=+
  Sum of Elements1 : Sum  Inputs=+
  Terminator : Terminator
  Terminator1 : Terminator
  Terminator2 : Terminator
  To Workspace : ToWorkspace  VariableName=u_pA  SampleTime=-1
  To Workspace1 : ToWorkspace  VariableName=u_aT  SampleTime=-1
  To Workspace3 : ToWorkspace  VariableName=dfcu_pa  SampleTime=-1
      settings: Save2DSignal=2-D array (concatenate along first dimension)
  To Workspace4 : ToWorkspace  VariableName=dfcu_at  SampleTime=-1
      settings: Save2DSignal=2-D array (concatenate along first dimension)
  To Workspace5 : ToWorkspace  VariableName=discrete_time  SampleTime=-1
  To Workspace6 : ToWorkspace  VariableName=plot_at1  SampleTime=-1
      settings: Save2DSignal=2-D array (concatenate along first dimension)
  To Workspace7 : ToWorkspace  VariableName=plot_UPa  SampleTime=-1
      settings: Save2DSignal=2-D array (concatenate along first dimension)
  Vectorized SteadyState : Subsystem  mask(Digital Hydraulics){Kv=DFCU.PA_Kv, dp_min=ptr}
      mask prompts: Kv "Orifice Flow Coefficient(s) [SI-units]:"; dp_min "min pressure differential [Pa] :"
      mask help:
      | Flow estimate by utilizing square root model only. Minimum pressure is
      | required to prevent infinities at dQ/dp state.
      |
      | Use scalar parameters model on/off-valve.
      | Use vector parameters model array of on/off-valves a.k.a DFCU
  Vectorized SteadyState1 : Subsystem  mask(Digital Hydraulics){Kv=DFCU.AT_Kv, dp_min=ptr}
      mask prompts: Kv "Orifice Flow Coefficient(s) [SI-units]:"; dp_min "min pressure differential [Pa] :"
      mask help:
      | Flow estimate by utilizing square root model only. Minimum pressure is
      | required to prevent infinities at dQ/dp state.
      |
      | Use scalar parameters model on/off-valve.
      | Use vector parameters model array of on/off-valves a.k.a DFCU
  Zero-Order Hold{,1..5} (6 alike) : ZeroOrderHold  SampleTime=Controller.ts
  Q_estimate : Outport
  uPA : Outport  Port=2
  uaT : Outport  Port=3
  State : Outport  Port=4
  Control_matrix : Outport  Port=5
  Con_PA : Outport  Port=6
  Con_AT : Outport  Port=7
  Q_PA : Outport  Port=8
  Q_AT : Outport  Port=9
  wires:
  Gain/1 -> Scope/1
  Data Type Conversion/1 -> State/1, Demux/1
  Zero-Order Hold4/1 -> Vectorized SteadyState1/2(p2)
  Minimum/1 -> Terminator1/1
  Demux/1 -> To Workspace/1, uPA/1, Gain2/1
  Sum of Elements1/1 -> To Workspace6/1
  Zero-Order Hold/1 -> Vectorized SteadyState/1(p1)
  Q_ref/1 -> Zero-Order Hold2/1
  Data Type Conversion1/1 -> Q_estimate/1
  Matrix Multiply/1 -> Subtract/2, Selector2/1, Gain/1
  Vectorized SteadyState1/2(Q2) -> Terminator2/1
  pA1/1 -> Zero-Order Hold3/1, Zero-Order Hold1/1
  Demux/2 -> To Workspace1/1, uaT/1, Gain3/1
  Vectorized SteadyState1/1(Q1) -> Q_AT/1, Mux/2
  pP/1 -> Zero-Order Hold/1
  Mux/1 -> Matrix Multiply/2
  Zero-Order Hold1/1 -> Vectorized SteadyState/2(p2)
  Selector1/1 -> Data Type Conversion/1
  pT/1 -> Zero-Order Hold4/1
  Gain2/1 -> To Workspace3/1, Sum of Elements/1
  Vectorized SteadyState/1(Q1) -> Terminator/1
  Zero-Order Hold2/1 -> Subtract/1
  Vectorized SteadyState/2(Q2) -> Q_PA/1, Mux/1
  Gain3/1 -> To Workspace4/1, Sum of Elements1/1
  Digital Clock/1 -> To Workspace5/1
  Zero-Order Hold3/1 -> Vectorized SteadyState1/1(p1)
  Sum of Elements/1 -> To Workspace7/1
  Minimum/2 -> Selector2/2, Scope1/1, Selector1/2
  Add1/1 -> Minimum/1
  Selector2/1 -> Data Type Conversion1/1
  Subtract/1 -> Abs/1
  Control matrix/1 -> Con_AT/1, Con_PA/1, Control_matrix/1, Matrix Multiply/1, Selector1/1
  Abs/1 -> Gain1/1
  Switch_cost/1 -> Zero-Order Hold5/1
  Gain1/1 -> Add1/1
  Min/1 -> Add1/2
  Zero-Order Hold5/1 -> Add1/3

== system digiex3/MBC/mbc_PA/SWITCHING COST ==
  note: SWITCHING COST
  STATE : Inport
  CONTROL_MATRIX : Inport  Port=2
  Gain7 : Gain  Gain=switch_gain
  Logical Operator1 : Logic  Operator=XOR  AllPortsSameDT=off  OutDataTypeStr=boolean
  Matrix Multiply3 : Product  Multiplication=Matrix(*)
  Sum of Elements3 : Sum  Inputs=+
  Unit Delay1 : UnitDelay  SampleTime=Controller.ts
  ones vector : Constant  Value=DFCU.one
  MINIMUM : Outport
  wires:
  Matrix Multiply3/1 -> Logical Operator1/2
  ones vector/1 -> Matrix Multiply3/1
  Sum of Elements3/1 -> Gain7/1
  Logical Operator1/1 -> Sum of Elements3/1
  Gain7/1 -> MINIMUM/1
  Unit Delay1/1 -> Matrix Multiply3/2
  STATE/1 -> Unit Delay1/1
  CONTROL_MATRIX/1 -> Logical Operator1/1

== system digiex3/VALVE SYSTEM/AT-DFCU. /Polynomial flow equation ==
  In1 : Inport
  In2 : Inport  Port=2
  Constant : Constant  Value=3
  Gain : Gain  Gain=1/ptr
  Gain1 : Gain  Gain=0.5/sqrt(ptr)
  Product : Product  RndMeth=Zero
  Product1 : Product  RndMeth=Zero
  Sum : Sum  Inputs=|-+
  Out1 : Outport
  wires:
  In1/1 -> Gain/1, Product/2
  Gain/1 -> Sum/1
  Constant/1 -> Sum/2
  In2/1 -> Product/1
  Product/1 -> Gain1/1
  Sum/1 -> Product1/2
  Gain1/1 -> Product1/1
  Product1/1 -> Out1/1

== system digiex3/VALVE SYSTEM/PA-DFCU/Polynomial flow equation ==
  In1 : Inport
  In2 : Inport  Port=2
  Constant : Constant  Value=3
  Gain : Gain  Gain=1/ptr
  Gain1 : Gain  Gain=0.5/sqrt(ptr)
  Product : Product  RndMeth=Zero
  Product1 : Product  RndMeth=Zero
  Sum : Sum  Inputs=|-+
  Out1 : Outport
  wires:
  Product1/1 -> Out1/1
  Gain1/1 -> Product1/1
  Sum/1 -> Product1/2
  Product/1 -> Gain1/1
  In2/1 -> Product/1
  Constant/1 -> Sum/2
  Gain/1 -> Sum/1
  In1/1 -> Product/2, Gain/1

== system digiex3/VALVE SYSTEM/port oifice/Polynomial flow equation ==
  In1 : Inport
  In2 : Inport  Port=2
  Constant : Constant  Value=3
  Gain : Gain  Gain=1/ptr
  Gain1 : Gain  Gain=0.5/sqrt(ptr)
  Product : Product  RndMeth=Zero
  Product1 : Product  RndMeth=Zero
  Sum : Sum  Inputs=|-+
  Out1 : Outport
  wires:
  Product1/1 -> Out1/1
  Gain1/1 -> Product1/1
  Sum/1 -> Product1/2
  Product/1 -> Gain1/1
  In2/1 -> Product/1
  Constant/1 -> Sum/2
  Gain/1 -> Sum/1
  In1/1 -> Product/2, Gain/1

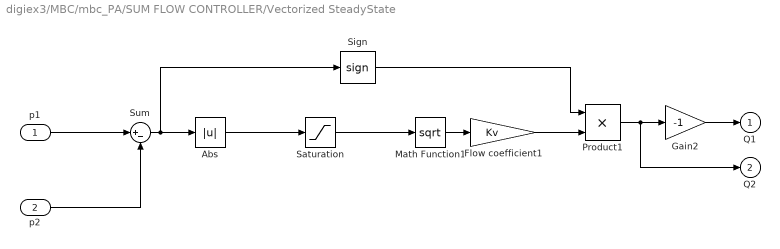
== system digiex3/MBC/mbc_PA/SUM FLOW CONTROLLER/Vectorized SteadyState ==
  p1 : Inport
  p2 : Inport  Port=2
  Abs : Abs  ZeroCross=off  SaturateOnIntegerOverflow=on
  Flow coefficient1 : Gain  Gain=Kv  SaturateOnIntegerOverflow=on  OutDataTypeStr=Inherit: Same as input  ParamDataTypeStr=Inherit: Same as input
  Gain2 : Gain  Gain=-1  SaturateOnIntegerOverflow=on  OutDataTypeStr=Inherit: Same as input  ParamDataTypeStr=Inherit: Same as input
  Math Function1 : Math  Operator=sqrt  SaturateOnIntegerOverflow=on
  Product1 : Product  SaturateOnIntegerOverflow=on  InputSameDT=on  OutDataTypeStr=Inherit: Same as first input
  Saturation : Saturate  UpperLimit=inf  LowerLimit=dp_min
  Sign : Signum  ZeroCross=off
  Sum : Sum  Inputs=|+-
  Q1 : Outport  InitialOutput=0
  Q2 : Outport  Port=2  InitialOutput=0
  wires:
  Gain2/1 -> Q1/1
  Sum/1 -> Abs/1, Sign/1
  Math Function1/1 -> Flow coefficient1/1
  Abs/1 -> Saturation/1
  Sign/1 -> Product1/1
  Product1/1 -> Q2/1, Gain2/1
  Flow coefficient1/1 -> Product1/2
  p1/1 -> Sum/1
  p2/1 -> Sum/2
  Saturation/1 -> Math Function1/1

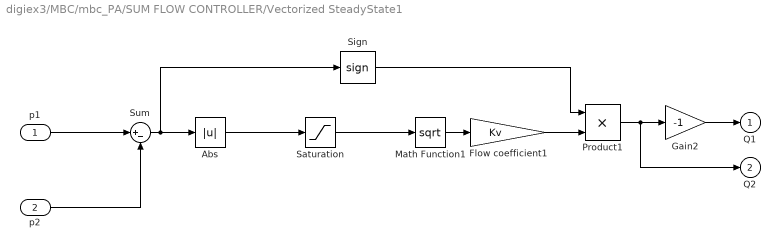
== system digiex3/MBC/mbc_PA/SUM FLOW CONTROLLER/Vectorized SteadyState1 ==
  p1 : Inport
  p2 : Inport  Port=2
  Abs : Abs  ZeroCross=off  SaturateOnIntegerOverflow=on
  Flow coefficient1 : Gain  Gain=Kv  SaturateOnIntegerOverflow=on  OutDataTypeStr=Inherit: Same as input  ParamDataTypeStr=Inherit: Same as input
  Gain2 : Gain  Gain=-1  SaturateOnIntegerOverflow=on  OutDataTypeStr=Inherit: Same as input  ParamDataTypeStr=Inherit: Same as input
  Math Function1 : Math  Operator=sqrt  SaturateOnIntegerOverflow=on
  Product1 : Product  SaturateOnIntegerOverflow=on  InputSameDT=on  OutDataTypeStr=Inherit: Same as first input
  Saturation : Saturate  UpperLimit=inf  LowerLimit=dp_min
  Sign : Signum  ZeroCross=off
  Sum : Sum  Inputs=|+-
  Q1 : Outport  InitialOutput=0
  Q2 : Outport  Port=2  InitialOutput=0
  wires:
  Saturation/1 -> Math Function1/1
  p2/1 -> Sum/2
  p1/1 -> Sum/1
  Flow coefficient1/1 -> Product1/2
  Product1/1 -> Gain2/1, Q2/1
  Sign/1 -> Product1/1
  Abs/1 -> Saturation/1
  Math Function1/1 -> Flow coefficient1/1
  Sum/1 -> Sign/1, Abs/1
  Gain2/1 -> Q1/1
